simulink model "MPC_point_6"  (R2022a)
settings: Solver=VariableStepAuto  StartTime=0.0  StopTime=10.0  RelTol=1e-3
values from neighbouring files (symbols this model uses):
  C = [0       1      0  0 ... (first row only)    [main.m]
  C_states = eye(length(A))    [main.m]
  D_states = zeros(length(B), 1)    [main.m]
  N5 = 100    [main.m]
  Q5 = Q_d    [main.m]
  R5 = R_d    (= 10000)    [main.m]
  S5 = P_d    [main.m]
  sysd = c2d(sys,T_sampling)    [main.m]
  T_sampling = 2*pi/omega_sampling    [main.m]
  u_max = deg2rad(15)    [main.m]
  u_min = deg2rad(-15)    [main.m]
  x0 = [deg2rad(0) deg2rad(15) 0 -300]    [main.m]
  x2_max = deg2rad(20)    [main.m]
  x2_min = deg2rad(-20)    [main.m]
  x_ref = [0 0 0 0]    [main.m]
undefined symbols (not defined in the file or in its folder): Klqr_d, mpc_point_3, mpc_point_5, mpc_point_6, over_shot_constraint
settings Model: Creator=g_mor  LastModifiedBy=g_mor

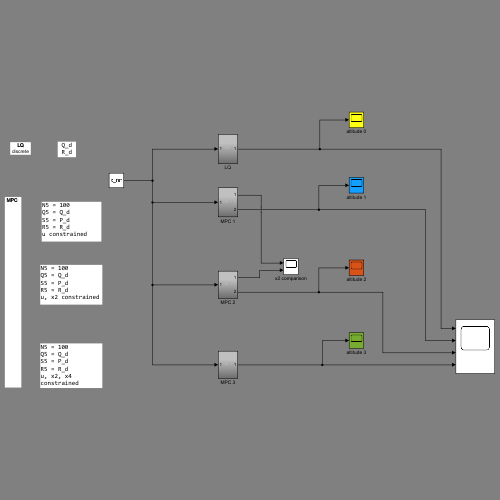
[thumbnail: Simulink's stored preview of the top-level diagram]
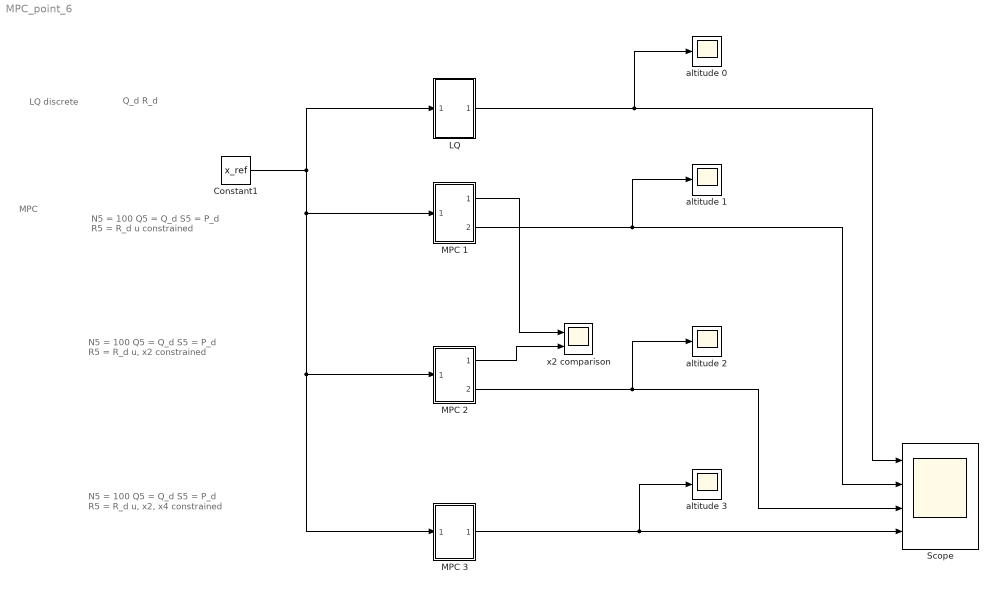
== system MPC_point_6 ==
  note: N5 = 100
      | Q5 = Q_d
      | S5 = P_d
      | R5 = R_d
      | u, x2 constrained
  note: LQ
      | discrete
  note: MPC
  note: Q_d
      | R_d
  note: N5 = 100
      | Q5 = Q_d
      | S5 = P_d
      | R5 = R_d
      | u constrained
  note: N5 = 100
      | Q5 = Q_d
      | S5 = P_d
      | R5 = R_d
      | u, x2, x4 constrained
  Constant1 : Constant  Value=x_ref
  LQ : Subsystem
  MPC 1 : Subsystem
  MPC 2 : Subsystem
  MPC 3 : Subsystem
  Scope : Scope  NumInputPorts=4
  altitude {0..3} (4 alike) : Scope
  x2 comparison : Scope  NumInputPorts=2
  wires:
  MPC 2/1(Out1) -> x2 comparison/2
  MPC 1/2(Out2) -> Scope/2, altitude 1/1
  LQ/1(Out1) -> altitude 0/1, Scope/1
  MPC 2/2(Out2) -> altitude 2/1, Scope/3
  MPC 1/1(Out1) -> x2 comparison/1
  Constant1/1 -> MPC 3/1(In1), MPC 2/1(In1), MPC 1/1(In1), LQ/1(In1)
  MPC 3/1(Out1) -> altitude 3/1, Scope/4

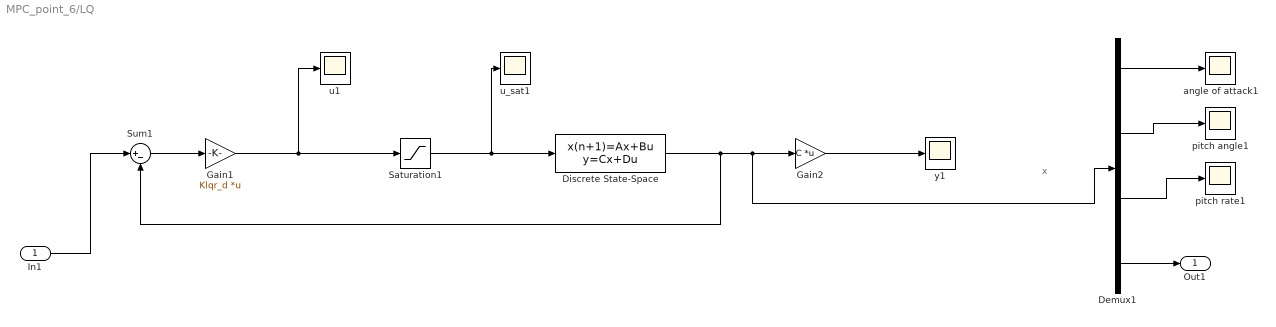
== system MPC_point_6/LQ ==
  note: x
  In1 : Inport
  Demux1 : Demux
  Discrete State-Space : DiscreteStateSpace  A=sysd.A  B=sysd.B  C=C_states  D=D_states  InitialCondition=x0  SampleTime=T_sampling
  Gain1 : Gain  Gain=Klqr_d  Multiplication=Matrix(K*u)
  Gain2 : Gain  Gain=C  Multiplication=Matrix(K*u)
  Saturation1 : Saturate  UpperLimit=u_max  LowerLimit=u_min
  Sum1 : Sum  Inputs=|+-
  angle of attack1 : Scope
  pitch angle1 : Scope
  pitch rate1 : Scope
  u1 : Scope
  u_sat1 : Scope
  y1 : Scope
  Out1 : Outport
  wires:
  Gain2/1 -> y1/1
  Discrete State-Space/1 -> Demux1/1, Gain2/1, Sum1/2
  Saturation1/1 -> Discrete State-Space/1, u_sat1/1
  Gain1/1 -> u1/1, Saturation1/1
  Demux1/4 -> Out1/1
  Demux1/1 -> angle of attack1/1
  Sum1/1 -> Gain1/1
  Demux1/2 -> pitch angle1/1
  Demux1/3 -> pitch rate1/1
  In1/1 -> Sum1/1

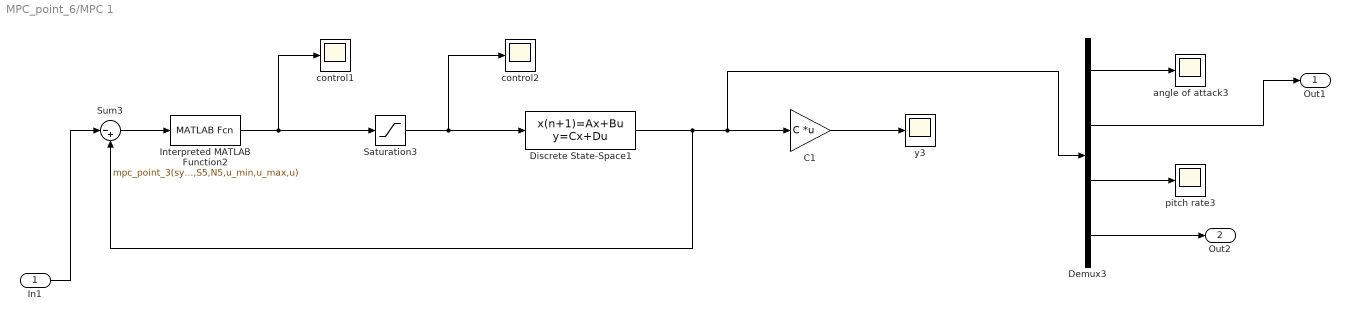
== system MPC_point_6/MPC 1 ==
  In1 : Inport
  C1 : Gain  Gain=C  Multiplication=Matrix(K*u)
  Demux3 : Demux
  Discrete State-Space1 : DiscreteStateSpace  A=sysd.A  B=sysd.B  C=C_states  D=D_states  InitialCondition=x0  SampleTime=T_sampling
  Interpreted MATLAB Function2 : MATLABFcn  MATLABFcn=mpc_point_3(sysd.A,sysd.B,Q5,R5,S5,N5,u_min,u_max,u)  OutputDimensions=1
  Saturation3 : Saturate  UpperLimit=u_max  LowerLimit=u_min
  Sum3 : Sum  Inputs=|-+
  angle of attack3 : Scope
  control1 : Scope
  control2 : Scope
  pitch rate3 : Scope
  y3 : Scope
  Out1 : Outport
  Out2 : Outport  Port=2
  wires:
  C1/1 -> y3/1
  Interpreted MATLAB Function2/1 -> Saturation3/1, control1/1
  Demux3/1 -> angle of attack3/1
  Discrete State-Space1/1 -> C1/1, Demux3/1, Sum3/2
  Demux3/4 -> Out2/1
  Saturation3/1 -> Discrete State-Space1/1, control2/1
  Sum3/1 -> Interpreted MATLAB Function2/1
  Demux3/3 -> pitch rate3/1
  In1/1 -> Sum3/1
  Demux3/2 -> Out1/1

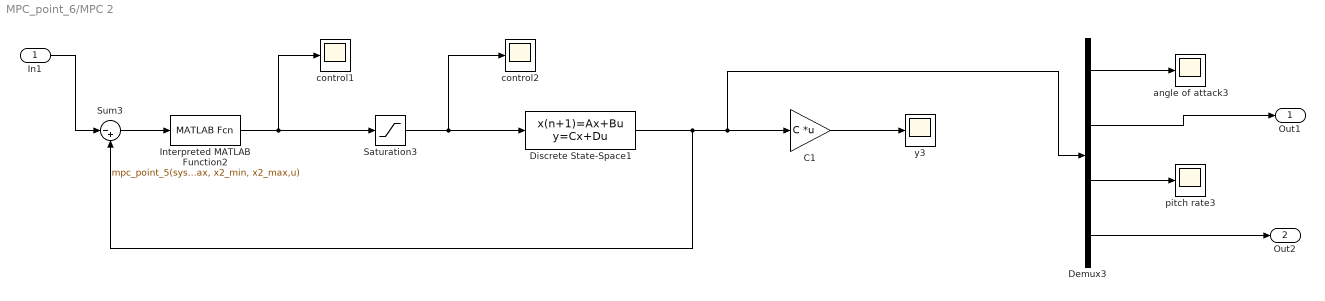
== system MPC_point_6/MPC 2 ==
  In1 : Inport
  C1 : Gain  Gain=C  Multiplication=Matrix(K*u)
  Demux3 : Demux
  Discrete State-Space1 : DiscreteStateSpace  A=sysd.A  B=sysd.B  C=C_states  D=D_states  InitialCondition=x0  SampleTime=T_sampling
  Interpreted MATLAB Function2 : MATLABFcn  MATLABFcn=mpc_point_5(sysd.A,sysd.B,Q5,R5,S5,N5,u_min,u_max, x2_min, x2_max,u)  OutputDimensions=1
  Saturation3 : Saturate  UpperLimit=u_max  LowerLimit=u_min
  Sum3 : Sum  Inputs=|-+
  angle of attack3 : Scope
  control1 : Scope
  control2 : Scope
  pitch rate3 : Scope
  y3 : Scope
  Out1 : Outport
  Out2 : Outport  Port=2
  wires:
  Interpreted MATLAB Function2/1 -> Saturation3/1, control1/1
  Demux3/1 -> angle of attack3/1
  Saturation3/1 -> Discrete State-Space1/1, control2/1
  Sum3/1 -> Interpreted MATLAB Function2/1
  C1/1 -> y3/1
  Demux3/3 -> pitch rate3/1
  Discrete State-Space1/1 -> C1/1, Demux3/1, Sum3/2
  In1/1 -> Sum3/1
  Demux3/2 -> Out1/1
  Demux3/4 -> Out2/1

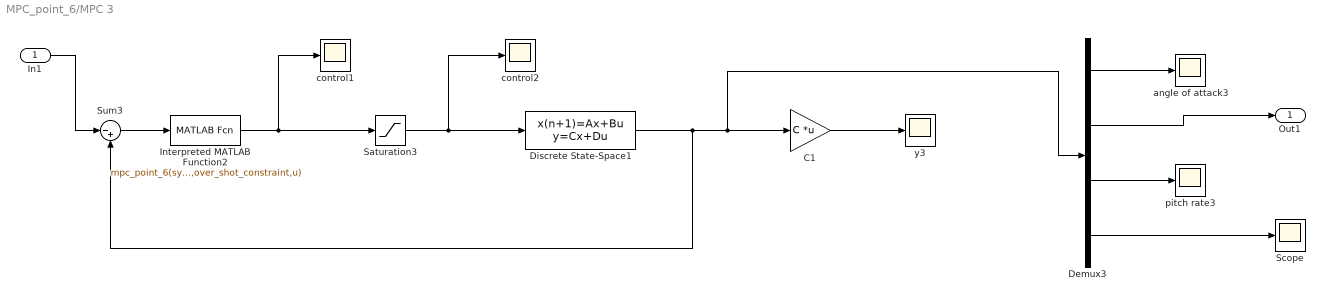
== system MPC_point_6/MPC 3 ==
  In1 : Inport
  C1 : Gain  Gain=C  Multiplication=Matrix(K*u)
  Demux3 : Demux
  Discrete State-Space1 : DiscreteStateSpace  A=sysd.A  B=sysd.B  C=C_states  D=D_states  InitialCondition=x0  SampleTime=T_sampling
  Interpreted MATLAB Function2 : MATLABFcn  MATLABFcn=mpc_point_6(sysd.A,sysd.B,Q5,R5,S5,N5,u_min,u_max, x2_min, x2_max,x0,over_shot_constraint,u)  OutputDimensions=1
  Saturation3 : Saturate  UpperLimit=u_max  LowerLimit=u_min
  Scope : Scope
  Sum3 : Sum  Inputs=|-+
  angle of attack3 : Scope
  control1 : Scope
  control2 : Scope
  pitch rate3 : Scope
  y3 : Scope
  Out1 : Outport
  wires:
  Interpreted MATLAB Function2/1 -> Saturation3/1, control1/1
  Demux3/1 -> angle of attack3/1
  Saturation3/1 -> Discrete State-Space1/1, control2/1
  Sum3/1 -> Interpreted MATLAB Function2/1
  C1/1 -> y3/1
  Demux3/3 -> pitch rate3/1
  Discrete State-Space1/1 -> C1/1, Demux3/1, Sum3/2
  In1/1 -> Sum3/1
  Demux3/2 -> Out1/1
  Demux3/4 -> Scope/1
